simulink model "SST_Basic_Model"  (R2025b)
settings: Solver=ode45  StartTime=0.0  StopTime=0.2  MaxStep=1e-5  RelTol=1e-4
libraries: slpidlib x1, simulink x1

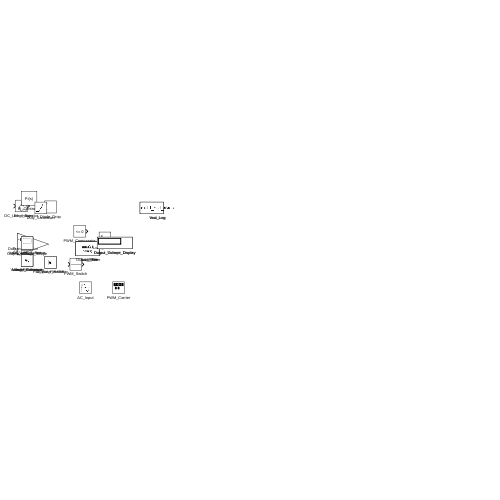
[thumbnail: Simulink's stored preview of the top-level diagram]
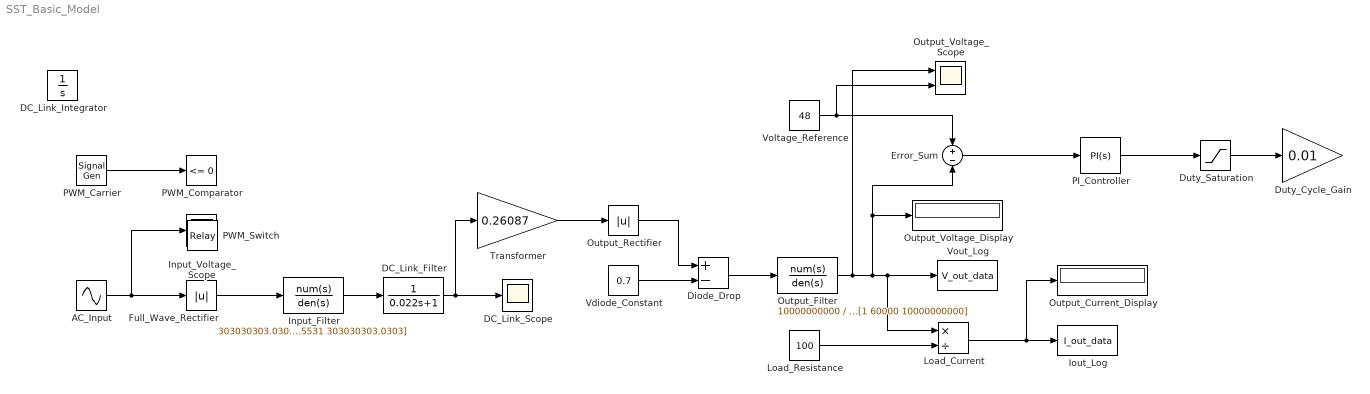
== system SST_Basic_Model ==
  AC_Input : Sin  Amplitude=325.2691  Frequency=314.1593  SampleTime=0
  DC_Link_Filter : TransferFcn  Numerator=1  Denominator=[0.022 1]
  DC_Link_Integrator : Integrator  InitialCondition=292.7422
  DC_Link_Scope : Scope
  Diode_Drop : Sum  Inputs=+-
  Duty_Cycle_Gain : Gain  Gain=0.01
  Duty_Saturation : Saturate  UpperLimit=0.95  LowerLimit=0.05
  Error_Sum : Sum  Inputs=+-
  Full_Wave_Rectifier : Abs  SaturateOnIntegerOverflow=off
  Input_Filter : TransferFcn  Numerator=303030303.0303  Denominator=[1 3481.5531 303030303.0303]
  Input_Voltage_Scope : Scope
  Iout_Log : ToWorkspace  VariableName=I_out_data  SaveFormat=Timeseries  SampleTime=-1
  Load_Current : Product  Inputs=*/
  Load_Resistance : Constant  Value=100
  Output_Current_Display : Display
  Output_Filter : TransferFcn  Numerator=10000000000  Denominator=[1 60000 10000000000]
  Output_Rectifier : Abs  SaturateOnIntegerOverflow=off
  Output_Voltage_Display : Display
  Output_Voltage_Scope : Scope  NumInputPorts=2
  PI_Controller : slpidlib/PID Controller  Controller=PI  Form=Parallel  TimeDomain=Continuous-time  UseExternalTs=off  SampleTime=-1  IntegratorMethod=Forward Euler  FilterMethod=Forward Euler  ControllerParametersSource=internal  P=0.5  I=10  UseKiTs=off  D=0  UseExternalDerivativeSource=off  N=100  UseFilter=on  TunerSelectOption=Transfer Function Based (PID Tuner App)  InitialConditionSource=internal  InitialConditionForIntegrator=0  InitialConditionForFilter=0  DifferentiatorICPrevScaledInput=0  ExternalReset=none  TrackingMode=off  Kt=1  LimitOutput=off  SatLimitsSource=internal  UpperSaturationLimit=inf  LowerSaturationLimit=-inf  LinearizeAsGain=on  AntiWindupMode=none  Kb=1  LimitIntegrator=off  UpperIntegratorSaturationLimit=inf  LowerIntegratorSaturationLimit=-inf  POutMin=[]  POutMax=[]  IOutMin=[]  IOutMax=[]  DOutMin=[]  DOutMax=[]  NOutMin=[]  NOutMax=[]  SumOutMin=[]  SumOutMax=[]  SaturationOutMin=[]  SaturationOutMax=[]  PParamMin=[]  PParamMax=[]  IParamMin=[]  IParamMax=[]  DParamMin=[]  DParamMax=[]  NParamMin=[]  NParamMax=[]  KbParamMin=[]  KbParamMax=[]  KtParamMin=[]  KtParamMax=[]  KbOutMin=[]  KbOutMax=[]  KtOutMin=[]  KtOutMax=[]  IntegratorOutMin=[]  IntegratorOutMax=[]  FilterOutMin=[]  FilterOutMax=[]  SumI1OutMin=[]  SumI1OutMax=[]  SumI2OutMin=[]  SumI2OutMax=[]  SumI3OutMin=[]  SumI3OutMax=[]  SumI4OutMin=[]  SumI4OutMax=[]  SumDOutMin=[]  SumDOutMax=[]  DifferentiatorOutMin=[]  DifferentiatorOutMax=[]  FilterDiffOutCoefMin=[]  FilterDiffOutCoefMax=[]  ReciprocalOutMin=[]  ReciprocalOutMax=[]  SumDenOutMin=[]  SumDenOutMax=[]  SumNumOutMin=[]  SumNumOutMax=[]  DivideOutMin=[]  DivideOutMax=[]  UdiffTsProdOutMin=[]  UdiffTsProdOutMax=[]  NTsProdOutMin=[]  NTsProdOutMax=[]  UintegralTsProdOutMin=[]  UintegralTsProdOutMax=[]  UngainTsProdOutMin=[]  UngainTsProdOutMax=[]  ClampingZeroOutDataTypeStr=Inherit: Inherit via back propagation  ClampingZeroOutMin=[]  ClampingZeroOutMax=[]  FilterDenConstantOutDataTypeStr=Inherit: Inherit via back propagation  FilterDenConstantOutMin=[]  FilterDenConstantOutMax=[]  PCopyOutDataTypeStr=Inherit: Inherit via back propagation  PCopyOutMin=[]  PCopyOutMax=[]  NCopyOutDataTypeStr=Inherit: Inherit via back propagation  NCopyOutMin=[]  NCopyOutMax=[]  IntegratorContinuousStateAttributes=''  IntegratorStateMustResolveToSignalObject=off  IntegratorRTWStateStorageClass=Auto  FilterContinuousStateAttributes=''  FilterStateMustResolveToSignalObject=off  FilterRTWStateStorageClass=Auto  ParallelPVariant=InternalParameters  IdealPVariant=Disabled  IVariant=InternalParameters  DVariant=Disabled  IntegratorVariant=Continuous  SatVariant=Disabled  AWVariant=Passthrough  PCopyVariant=Disabled  TRVariant=Disabled  FdbkBlocksVariant=Forward  IdealPFdbkVariant=Disabled  SatFdbkVariant=Disabled  DerivativeFilterVariant=Disabled  NVariant=Disabled  NCopyVariant=Disabled_SignalSpec  FilterICVariant=Disabled  IntegratorICVariant=InternalICs  ExternalResetVariant=Disabled  TRSumVariant=Passthrough  SumFdbkVariant=Disabled  SumVariant=Sum_PI  TsampFilterVariant=InternalTs  TsampNgainVariant=Passthrough  TsampIntegralVariant=Disabled_SignalSpec  ExternalSaturationOutDataTypeStr=Inherit: Same as second input  DerivativeSourceVariant=Disabled  PreIntVariant=InternalPreInt
  PWM_Carrier : SignalGenerator  WaveForm=sawtooth  Frequency=100000  Units=rad/sec
  PWM_Comparator : simulink/Logic and Bit Operations/Compare To Zero  relop=<=  OutDataTypeStr=boolean
  PWM_Switch : Relay  OnSwitchValue=0.01  OffSwitchValue=-0.01
  Transformer : Gain  Gain=0.26087
  Vdiode_Constant : Constant  Value=0.7
  Voltage_Reference : Constant  Value=48
  Vout_Log : ToWorkspace  VariableName=V_out_data  SaveFormat=Timeseries  SampleTime=-1
  wires:
  Duty_Saturation/1 -> Duty_Cycle_Gain/1
  PI_Controller/1 -> Duty_Saturation/1
  Load_Current/1 -> Iout_Log/1, Output_Current_Display/1
  AC_Input/1 -> Input_Voltage_Scope/1, Full_Wave_Rectifier/1
  Full_Wave_Rectifier/1 -> Input_Filter/1
  Input_Filter/1 -> DC_Link_Filter/1
  Diode_Drop/1 -> Output_Filter/1
  Vdiode_Constant/1 -> Diode_Drop/2
  PWM_Carrier/1 -> PWM_Comparator/1
  Voltage_Reference/1 -> Output_Voltage_Scope/2, Error_Sum/1
  Error_Sum/1 -> PI_Controller/1
  Transformer/1 -> Output_Rectifier/1
  Output_Rectifier/1 -> Diode_Drop/1
  Output_Filter/1 -> Vout_Log/1, Load_Current/1, Output_Voltage_Display/1, Error_Sum/2, Output_Voltage_Scope/1
  DC_Link_Filter/1 -> DC_Link_Scope/1, Transformer/1
  Load_Resistance/1 -> Load_Current/2
